simulink model "CT_T1_Calibration_Modified"  (R2018a)
settings: Solver=ode1  StartTime=0.0  StopTime=500  FixedStep=0.1  RelTol=1e-3
undefined symbols (not defined in the file): Advantech, PCI
libraries: sldrtlib x2
settings Model: SimulationMode=external  ExtModeTrigDuration=60000  ExtModeArchiveMode=auto  ExtModeArchiveFileName=data  ExtModeArchiveDirName=c:\users\Warren\  ExtModeAddSuffixToVar=on  Creator=Erkan Zergeroglu  LastModifiedBy=adonnel7
settings DataIOCC: Decimation=10  SaveFinalState=on  SaveFormat=StructureWithTime  SignalLoggingSaveFormat=ModelDataLogs  SaveState=on
settings OptimizationCC: BlockReduction=off  BooleanDataType=off  ExpressionDepthLimit=2147483647  InitFltsAndDblsToZero=on
settings DebuggingCC: SaveWithParameterizedLinksMsg=none  UnderspecifiedInitializationDetection=Classic  MergeDetectMultiDrivingBlocksExec=none  SignalResolutionControl=TryResolveAllWithWarning  MultiTaskDSMMsg=warning  MultiTaskCondExecSysMsg=none  FcnCallInpInsideContextMsg=warning  StateNameClashWarn=warning  SFUnexpectedBacktrackingDiag=warning  SFNoUnconditionalDefaultTransitionDiag=warning  SFExecutionAtInitializationDiag=none
settings ModelReferenceCC: PropagateSignalLabelsOutOfModel=off
settings RTWCC: SystemTargetFile=sldrt.tlc  TemplateMakefile=sldrt.tmf  Description=Simulink Desktop Real-Time  RTWCompilerOptimization=on
settings CodeAppCC: MaxIdLength=95  StateflowObjectComments=on
settings SimulinkDesktopRealTimeCC: TargetPreCompLibLocation=C:\Program Files\MATLAB\R2018a\toolbox\sldrt\lib\win64  TargetLangStandard=C89/C90 (ANSI)  ModelReferenceCompliant=off  CompOptLevelCompliant=off  SupportVariableSizeSignals=off
settings ConfigComp: CovMetricSettings=dw  CovHtmlReporting=on  CovSaveCumulativeToWorkspaceVar=on  CovSaveSingleToWorkspaceVar=on  CovExternalEMLEnable=off

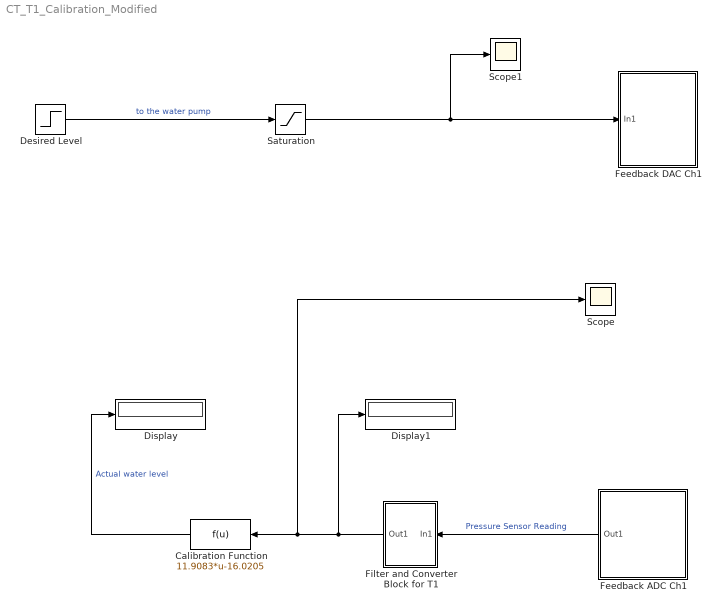
== system CT_T1_Calibration_Modified ==
  Calibration Function : Fcn  Expr=11.9083*u-16.0205
  Desired Level : Step  Time=0  After=0  SampleTime=0
  Display : Display
  Display1 : Display
  Feedback ADC Ch1 : Subsystem  mask{Tsamp=0.1}
      mask prompts: Tsamp "Sampling time"
      mask Display:
      | image(imread('bckg.bmp'))
      | disp('PCI1711 \n Lab I/O Board \n\n Feedback  ADC')
  Feedback DAC Ch1 : Subsystem  mask(DAC Unit for Feedback Experiments){st=0.1, ch=1}
      mask prompts: st "Sample Time"; ch "Output Channel"
      mask help:
      | Digital to Analog Output  for Feedback Experiments
      | using Advantech PCI1711  I/O board
      mask Display:
      | image(imread('bckg.bmp'))
      | disp('PCI1711 \n Lab I/O Board \n\n Feedback  DAC')
  Filter and Converter Block for T1 : Subsystem
      mask Display:
      | image(imread('bckg.bmp'))
      | disp('Filter \n & \n Converter')
  Saturation : Saturate  UpperLimit=4.5  LowerLimit=0
  Scope : Scope
  Scope1 : Scope
  wires:
  Feedback ADC Ch1/1(Out1) -> Filter and Converter Block for T1/1(In1)  "Pressure Sensor Reading"
  Desired Level/1 -> Saturation/1  "to the water pump"
  Calibration Function/1 -> Display/1  "Actual water level"
  Filter and Converter Block for T1/1(Out1) -> Display1/1, Scope/1, Calibration Function/1
  Saturation/1 -> Scope1/1, Feedback DAC Ch1/1(In1)

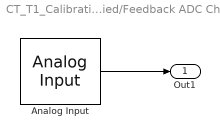
== system CT_T1_Calibration_Modified/Feedback ADC Ch1 ==
  Analog Input : sldrtlib/Analog Input  SampleTime=Tsamp  MaxMissedTicks=10  ShowMissedTicks=off  YieldWhenWaiting=off  DrvName=Advantech/PCI-1711  DrvAddress=4294967295  DrvOptions=zeros(1,0)  Channels=2  RangeMode=1  VoltRange=1  DataType=1
      settings: AttributesFormatString=Advantech\nPCI-1711 [auto]  SourceProductName=Simulink Desktop Real-Time
  Out1 : Outport
  wires:
  Analog Input/1 -> Out1/1

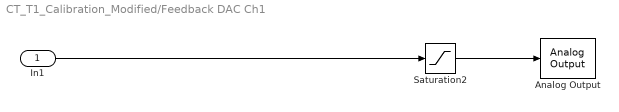
== system CT_T1_Calibration_Modified/Feedback DAC Ch1 ==
  In1 : Inport
  Analog Output : sldrtlib/Analog Output  SampleTime=st  MaxMissedTicks=10  ShowMissedTicks=off  YieldWhenWaiting=off  DrvName=Advantech/PCI-1711  DrvAddress=4294967295  DrvOptions=zeros(1,0)  Channels=ch  RangeMode=1  VoltRange=2  InitialValue=0  FinalValue=0
      settings: AttributesFormatString=Advantech\nPCI-1711 [auto]  SourceProductName=Simulink Desktop Real-Time
  Saturation2 : Saturate  UpperLimit=5  LowerLimit=0
  wires:
  In1/1 -> Saturation2/1
  Saturation2/1 -> Analog Output/1

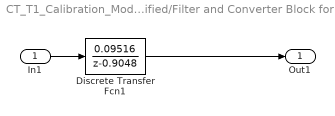
== system CT_T1_Calibration_Modified/Filter and Converter Block for T1 ==
  In1 : Inport
  Discrete Transfer Fcn1 : DiscreteTransferFcn  Numerator=[0.09516]  Denominator=[1 -0.9048]  SampleTime=0.1
  Out1 : Outport
  wires:
  In1/1 -> Discrete Transfer Fcn1/1
  Discrete Transfer Fcn1/1 -> Out1/1
